simulink model "adcs_plant"  (R2024b)
settings: Solver=ode4  StartTime=0.0  StopTime=30  FixedStep=0.01  RelTol=1e-3
model workspace (MAT data in the model file):
  J = [1  0  0; 0  2  0; 0  0  3]
  R_orbit = 6871000
  gyro_arw = 8.72664625997e-05
  gyro_bias_instab = 2.42406840555e-05
  k_stab = 1
  mu_earth = 398600441800000
libraries: simulink x2
settings Model: Creator=natha  LastModifiedBy=natha

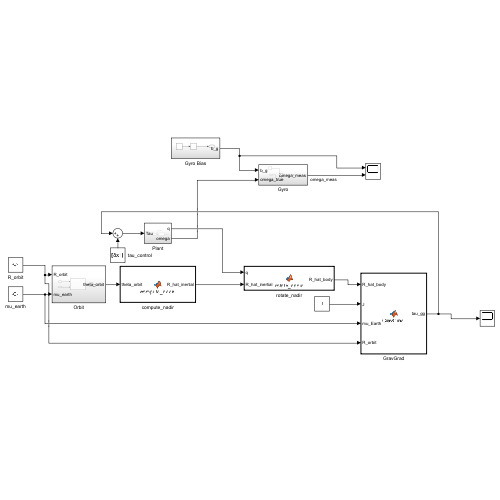
[thumbnail: Simulink's stored preview of the top-level diagram]
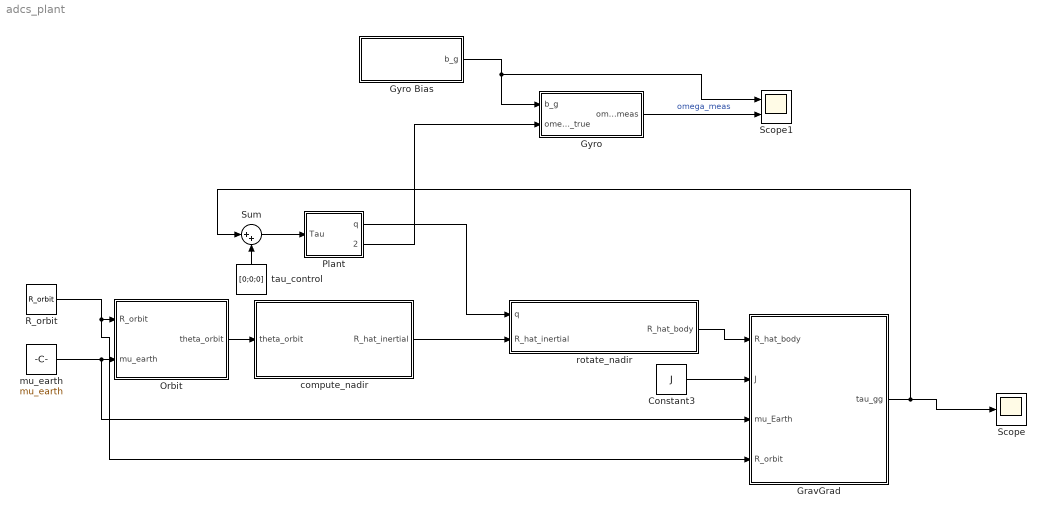
== system adcs_plant ==
  Constant3 : Constant  Value=J
  GravGrad : MATLAB Function  TreatAsAtomicUnit=on
  Gyro : Subsystem
  Gyro Bias : Subsystem
  Orbit : Subsystem
  Plant : Subsystem
  R_orbit : Constant  Value=R_orbit
  Scope : Scope
  Scope1 : Scope  NumInputPorts=2
  Sum : Sum  Inputs=|++
  compute_nadir : MATLAB Function  TreatAsAtomicUnit=on
  mu_earth : Constant  Value=mu_earth
  rotate_nadir : MATLAB Function  TreatAsAtomicUnit=on
  tau_control : Constant  Value=[0;0;0]
  wires:
  Sum/1 -> Plant/1(Tau)
  mu_earth/1 -> GravGrad/3(mu_Earth), Orbit/2(mu_earth)
  R_orbit/1 -> GravGrad/4(R_orbit), Orbit/1(R_orbit)
  Orbit/1(theta_orbit) -> compute_nadir/1(theta_orbit)
  Plant/1(q) -> rotate_nadir/1(q)
  compute_nadir/1(R_hat_inertial) -> rotate_nadir/2(R_hat_inertial)
  rotate_nadir/1(R_hat_body) -> GravGrad/1(R_hat_body)
  Constant3/1 -> GravGrad/2(J)
  tau_control/1 -> Sum/2
  GravGrad/1(tau_gg) -> Scope/1, Sum/1
  Plant/2(omega) -> Gyro/2(omega_true)
  Gyro Bias/1(b_g) -> Scope1/1, Gyro/1(b_g)
  Gyro/1(omega_meas) -> Scope1/2  "omega_meas"

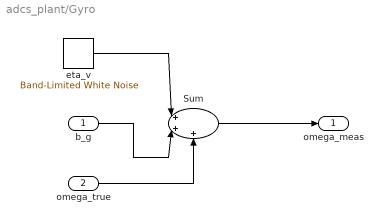
== system adcs_plant/Gyro ==
  b_g : Inport
  omega_true : Inport  Port=2
  Sum : Sum  Inputs=|+++
  eta_v : simulink/Sources/Band-Limited White Noise  Cov=gyro_arw^2  Ts=0.01  seed=[23341]
  omega_meas : Outport
  wires:
  eta_v/1 -> Sum/1
  b_g/1 -> Sum/2
  omega_true/1 -> Sum/3
  Sum/1 -> omega_meas/1

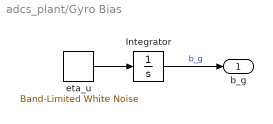
== system adcs_plant/Gyro Bias ==
  Integrator : Integrator  InitialCondition=2.4e-6
  eta_u : simulink/Sources/Band-Limited White Noise  Cov=(gyro_bias_instab/60)^2  Ts=0.1  seed=[23341]
  b_g : Outport
  wires:
  eta_u/1 -> Integrator/1
  Integrator/1 -> b_g/1  "b_g"

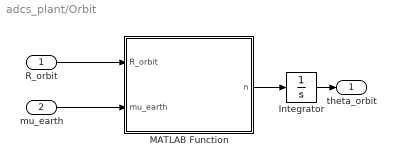
== system adcs_plant/Orbit ==
  R_orbit : Inport
  mu_earth : Inport  Port=2
  Integrator : Integrator
  MATLAB Function : MATLAB Function  TreatAsAtomicUnit=on
  theta_orbit : Outport
  wires:
  MATLAB Function/1(n) -> Integrator/1
  Integrator/1 -> theta_orbit/1
  mu_earth/1 -> MATLAB Function/2(mu_earth)
  R_orbit/1 -> MATLAB Function/1(R_orbit)

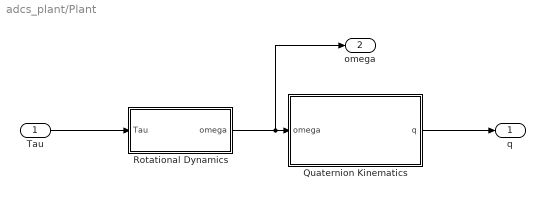
== system adcs_plant/Plant ==
  Tau : Inport
  Quaternion Kinematics : Subsystem
  Rotational Dynamics : Subsystem
  q : Outport
  omega : Outport  Port=2
  wires:
  Quaternion Kinematics/1(q) -> q/1
  Tau/1 -> Rotational Dynamics/1(Tau)
  Rotational Dynamics/1(omega) -> omega/1, Quaternion Kinematics/1(omega)

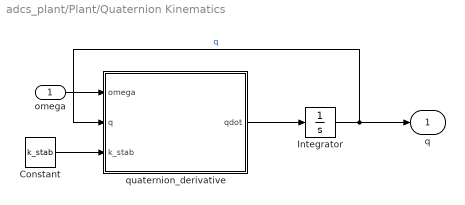
== system adcs_plant/Plant/Quaternion Kinematics ==
  omega : Inport  Unit=rad/s
  Constant : Constant  Value=k_stab
  Integrator : Integrator  InitialCondition=[0; 0; 0; 1]
  quaternion_derivative : MATLAB Function  TreatAsAtomicUnit=on
  q : Outport
  wires:
  quaternion_derivative/1(qdot) -> Integrator/1
  Integrator/1 -> q/1, quaternion_derivative/2(q)  "q"
  omega/1 -> quaternion_derivative/1(omega)
  Constant/1 -> quaternion_derivative/3(k_stab)

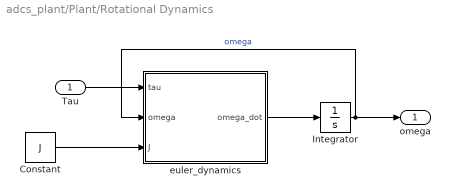
== system adcs_plant/Plant/Rotational Dynamics ==
  Tau : Inport  Unit=N*m
  Constant : Constant  Value=J
  Integrator : Integrator  InitialCondition=[0.01; 5; 0.01]
  euler_dynamics : MATLAB Function  TreatAsAtomicUnit=on
  omega : Outport  Unit=rad/s
  wires:
  Tau/1 -> euler_dynamics/1(tau)
  Constant/1 -> euler_dynamics/3(J)
  euler_dynamics/1(omega_dot) -> Integrator/1
  Integrator/1 -> euler_dynamics/2(omega), omega/1  "omega"

== matlab function adcs_plant/Plant/Rotational Dynamics/euler_dynamics ==
  data: tau input; omega_dot output; omega input; J input
function omega_dot = euler_dynamics(tau,omega,J)

omega_dot = J\(tau - cross(omega,J*omega));

== matlab function adcs_plant/Plant/Quaternion Kinematics/quaternion_derivative ==
  data: omega input; qdot output; q input; k_stab input
function qdot = quaternion_derivative(omega,q,k_stab)

Omega = [0 omega(3) -omega(2) omega(1);
         -omega(3) 0 omega(1) omega(2);
         omega(2) -omega(1) 0 omega(3);
         -omega(1) -omega(2) -omega(3) 0];


qdot = (1/2)*Omega*q + k_stab*(1 - q'*q)*q;

== matlab function adcs_plant/Orbit/MATLAB Function ==
  data: n output; R_orbit input; mu_earth input
function n = meanmotion(R_orbit,mu_earth)

n = sqrt(mu_earth/R_orbit^3);

== matlab function adcs_plant/compute_nadir ==
  data: theta_orbit input; R_hat_inertial output
function R_hat_inertial = compute_nadir(theta_orbit)

R_hat_inertial = [cos(theta_orbit); sin(theta_orbit); 0];

== matlab function adcs_plant/rotate_nadir ==
  data: q input; R_hat_body output; R_hat_inertial input
function R_hat_body = rotate_nadir(q,R_hat_inertial)

DCM = [1-2*(q(2)^2+q(3)^2) 2*(q(1)*q(2)+q(3)*q(4)) 2*(q(1)*q(3)-q(2)*q(4));
       2*(q(1)*q(2)-q(3)*q(4)) 1-2*(q(1)^2+q(3)^2) 2*(q(2)*q(3)+q(1)*q(4));
       2*(q(1)*q(3)+q(2)*q(4)) 2*(q(2)*q(3)-q(1)*q(4)) 1-2*(q(1)^2+q(2)^2)];

R_hat_body = DCM * R_hat_inertial;

== matlab function adcs_plant/GravGrad ==
  data: R_hat_body input; tau_gg output; J input; mu_Earth input; R_orbit input
function tau_gg = GravGrad(R_hat_body,J,mu_Earth,R_orbit)

tau_gg = (3*mu_Earth/R_orbit^3) * cross(R_hat_body,J*R_hat_body);
